simulink model "StepperMotor"  (R2020b)
settings: Solver=VariableStepAuto  StartTime=0.0  StopTime=10.0  RelTol=1e-3
values from neighbouring files (symbols this model uses):
  a1 = Beq + (ng* Kg^2 * nm* Kt * Km/Rm)    (= 0.07285017685)    [Lab4.m]
  a2 = Jeq    (= 0.002)    [Lab4.m]
  b = ng*Kg*nm*Kt/Rm    (= 0.1282365)    [Lab4.m]
  Kd = (2*zeta*wn*a2 - a1)/b    [Lab4.m]
  Kp = Kp - 8.5    [Lab4.m]
settings Model: Creator=17165  LastModifiedBy=gcola
settings DebuggingCC: SFMachineParentedDataDiag=error

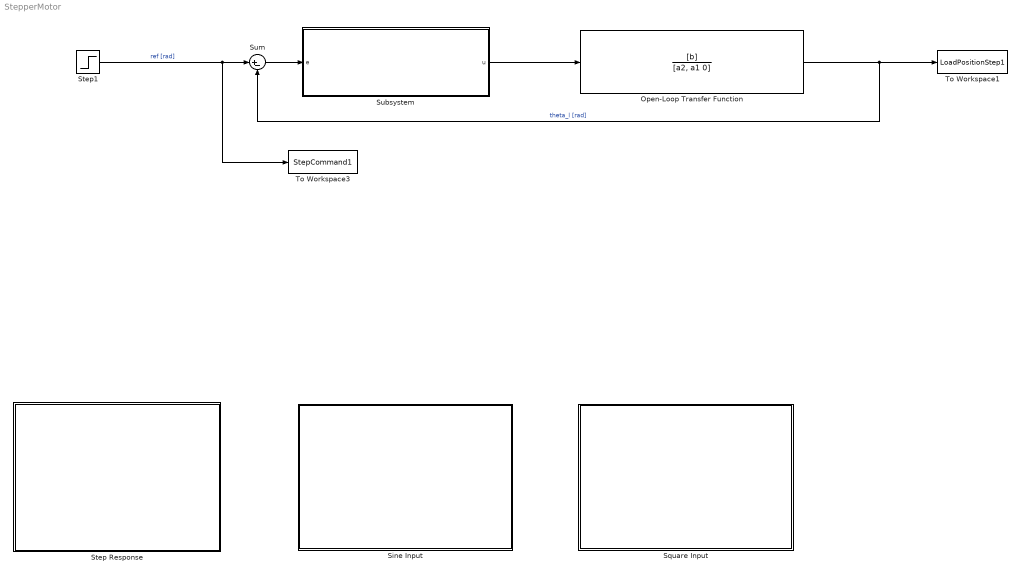
== system StepperMotor ==
  Open-Loop Transfer Function : TransferFcn  Numerator=[b]  Denominator=[a2, a1 0]
  Sine Input : Subsystem
  Square Input : Subsystem
  Step Response : Subsystem
  Step1 : Step  SampleTime=0
  Subsystem : Subsystem  mask{Kp=10, Kd=.1}
  Sum : Sum  Inputs=|+-
  To Workspace1 : ToWorkspace  VariableName=LoadPositionStep1  SampleTime=-1
  To Workspace3 : ToWorkspace  VariableName=StepCommand1  SampleTime=-1
  wires:
  Step1/1 -> Sum/1, To Workspace3/1  "ref [rad]"
  Open-Loop Transfer Function/1 -> Sum/2, To Workspace1/1  "theta_l [rad]"
  Sum/1 -> Subsystem/1(e)
  Subsystem/1(u) -> Open-Loop Transfer Function/1

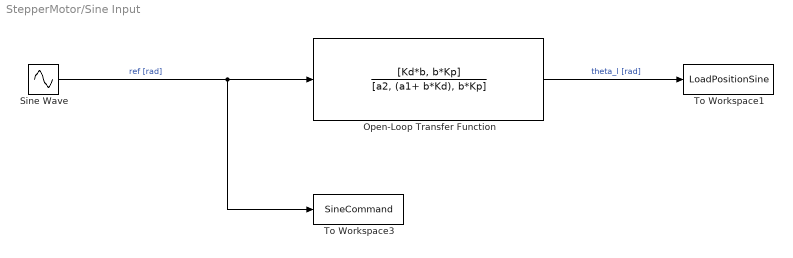
== system StepperMotor/Sine Input ==
  Open-Loop Transfer Function : TransferFcn  Numerator=[Kd*b, b*Kp]  Denominator=[a2, (a1+ b*Kd), b*Kp]
  Sine Wave : Sin  Frequency=5  SampleTime=0
  To Workspace1 : ToWorkspace  VariableName=LoadPositionSine  SampleTime=-1
  To Workspace3 : ToWorkspace  VariableName=SineCommand  SampleTime=-1
  wires:
  Sine Wave/1 -> To Workspace3/1, Open-Loop Transfer Function/1  "ref [rad]"
  Open-Loop Transfer Function/1 -> To Workspace1/1  "theta_l [rad]"

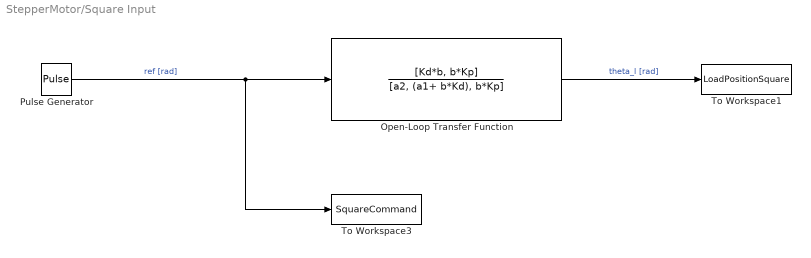
== system StepperMotor/Square Input ==
  Open-Loop Transfer Function : TransferFcn  Numerator=[Kd*b, b*Kp]  Denominator=[a2, (a1+ b*Kd), b*Kp]
  Pulse Generator : DiscretePulseGenerator  PulseType=Time based  Period=1  PulseWidth=50
  To Workspace1 : ToWorkspace  VariableName=LoadPositionSquare  SampleTime=-1
  To Workspace3 : ToWorkspace  VariableName=SquareCommand  SampleTime=-1
  wires:
  Pulse Generator/1 -> To Workspace3/1, Open-Loop Transfer Function/1  "ref [rad]"
  Open-Loop Transfer Function/1 -> To Workspace1/1  "theta_l [rad]"

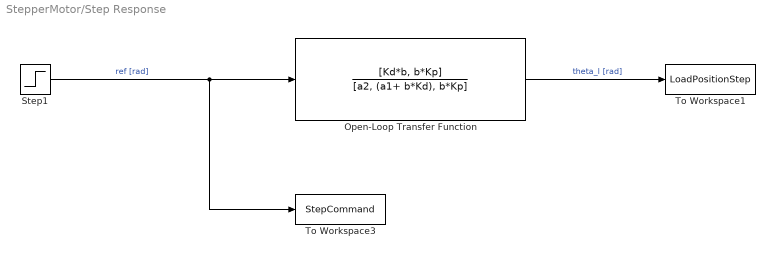
== system StepperMotor/Step Response ==
  Open-Loop Transfer Function : TransferFcn  Numerator=[Kd*b, b*Kp]  Denominator=[a2, (a1+ b*Kd), b*Kp]
  Step1 : Step  SampleTime=0
  To Workspace1 : ToWorkspace  VariableName=LoadPositionStep  SampleTime=-1
  To Workspace3 : ToWorkspace  VariableName=StepCommand  SampleTime=-1
  wires:
  Step1/1 -> To Workspace3/1, Open-Loop Transfer Function/1  "ref [rad]"
  Open-Loop Transfer Function/1 -> To Workspace1/1  "theta_l [rad]"

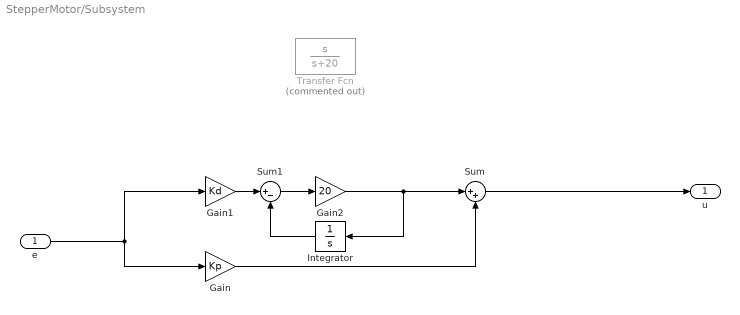
== system StepperMotor/Subsystem ==
  e : Inport
  Gain : Gain  Gain=Kp
  Gain1 : Gain  Gain=Kd
  Gain2 : Gain  Gain=20
  Integrator : Integrator
  Sum : Sum  Inputs=|++
  Sum1 : Sum  Inputs=|+-
  Transfer Fcn : TransferFcn  Commented=on  Numerator=[1 0]  Denominator=[1 20]
  u : Outport
  wires:
  e/1 -> Gain1/1, Gain/1
  Gain/1 -> Sum/2
  Sum/1 -> u/1
  Gain1/1 -> Sum1/1
  Sum1/1 -> Gain2/1
  Gain2/1 -> Integrator/1, Sum/1
  Integrator/1 -> Sum1/2
